simulink model "ThreeTank"  (R2020a)
settings: Solver=ode45  StartTime=0.0  StopTime=100  RelTol=1e-3
settings Model: Creator=gaoqiang  LastModifiedBy=bzhan
settings DataIOCC: SaveFormat=StructureWithTime
settings OptimizationCC: LifeSpan=inf
settings DebuggingCC: SFExecutionAtInitializationDiag=none  ArithmeticOperatorsInVariantConditions=warning
settings HardwareCC: ProdBitPerSizeT=32  ProdBitPerPtrDiffT=32  ProdWordSize=32  ProdHWDeviceType=Specified
settings SFSimCC: CustomCodeUndefinedFunction=UseInterfaceOnly
settings CodeAppCC: StateflowObjectComments=on

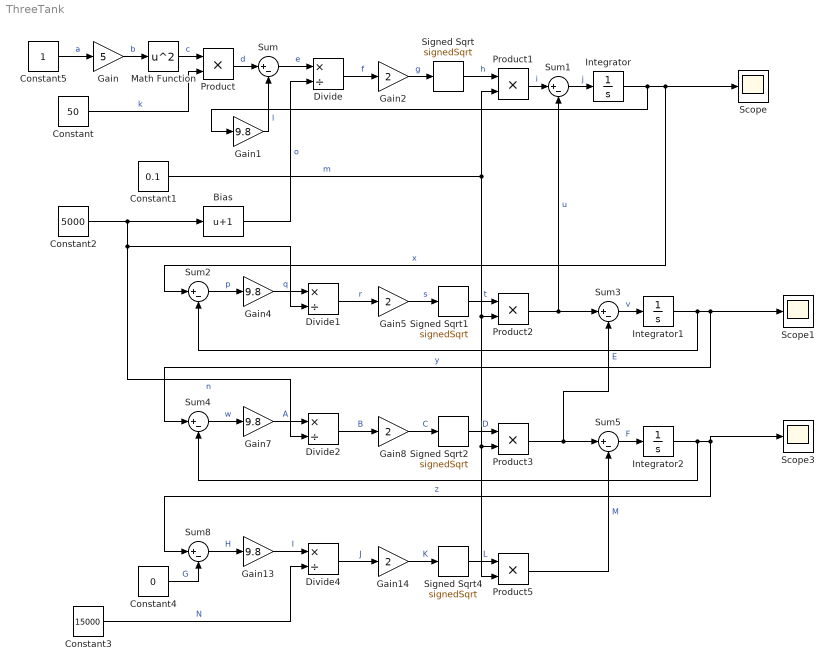
== system ThreeTank ==
  Bias : Bias  Bias=1
  Constant : Constant  Value=50
  Constant1 : Constant  Value=0.1
  Constant2 : Constant  Value=5000
  Constant3 : Constant  Value=15000
  Constant4 : Constant  Value=0
  Constant5 : Constant
  Divide{,1..2,4} (4 alike) : Product  Inputs=*/
  Gain : Gain  Gain=5
  Gain{1,4,7,13} (4 alike) : Gain  Gain=9.8
  Gain{2,5,8,14} (4 alike) : Gain  Gain=2
  Integrator : Integrator
  Integrator1 : Integrator
  Integrator2 : Integrator
  Math Function : Math  Operator=square  SignedPower=on  SaturateOnIntegerOverflow=on
  Product{,1..3,5} (5 alike) : Product
  Scope : Scope
  Scope1 : Scope
  Scope3 : Scope
  Signed Sqrt{,1..2,4} (4 alike) : Sqrt  Operator=signedSqrt  SaturateOnIntegerOverflow=on
  Sum{,1..5,8} (7 alike) : Sum  Inputs=|+-
  wires:
  Constant5/1 -> Gain/1  "a"
  Math Function/1 -> Product/1  "c"
  Gain/1 -> Math Function/1  "b"
  Constant/1 -> Product/2  "k"
  Gain1/1 -> Sum/2  "l"
  Product/1 -> Sum/1  "d"
  Sum/1 -> Divide/1  "e"
  Divide/1 -> Gain2/1  "f"
  Gain2/1 -> Signed Sqrt/1  "g"
  Signed Sqrt/1 -> Product1/1  "h"
  Product1/1 -> Sum1/1  "i"
  Sum1/1 -> Integrator/1  "j"
  Integrator/1 -> Scope/1, Sum2/1, Gain1/1  "x"
  Constant1/1 -> Product3/2, Product5/2, Product2/2, Product1/2  "m"
  Constant2/1 -> Divide2/2, Divide1/2, Bias/1  "n"
  Bias/1 -> Divide/2  "o"
  Sum2/1 -> Gain4/1  "p"
  Gain4/1 -> Divide1/1  "q"
  Divide1/1 -> Gain5/1  "r"
  Gain5/1 -> Signed Sqrt1/1  "s"
  Signed Sqrt1/1 -> Product2/1  "t"
  Product2/1 -> Sum3/1, Sum1/2  "u"
  Sum3/1 -> Integrator1/1  "v"
  Integrator1/1 -> Scope1/1, Sum4/1, Sum2/2  "y"
  Sum4/1 -> Gain7/1  "w"
  Product3/1 -> Sum3/2, Sum5/1  "E"
  Signed Sqrt2/1 -> Product3/1  "D"
  Gain7/1 -> Divide2/1  "A"
  Divide2/1 -> Gain8/1  "B"
  Gain8/1 -> Signed Sqrt2/1  "C"
  Integrator2/1 -> Scope3/1, Sum8/1, Sum4/2  "z"
  Sum5/1 -> Integrator2/1  "F"
  Sum8/1 -> Gain13/1  "H"
  Divide4/1 -> Gain14/1  "J"
  Gain13/1 -> Divide4/1  "I"
  Signed Sqrt4/1 -> Product5/1  "L"
  Gain14/1 -> Signed Sqrt4/1  "K"
  Product5/1 -> Sum5/2  "M"
  Constant3/1 -> Divide4/2  "N"
  Constant4/1 -> Sum8/2  "G"
